simulink model "mixing_tank"  (R2019b)
settings: Solver=FixedStepDiscrete  StartTime=0.0  StopTime=30.0  FixedStep=1  RelTol=1e-3  EnableMultiTasking=on
undefined symbols (not defined in the file): sigbuilder_block
settings Model: EnablePacing=on  PacingRate=0.500000  Creator=faaizz  LastModifiedBy=faaizz
settings SolverCC: AutoInsertRateTranBlk=on
settings DataIOCC: LimitDataPoints=on
settings OptimizationCC: LifeSpan=inf
settings DebuggingCC: AllowSymbolicDim=off  SFUnexpectedBacktrackingDiag=warning  SFNoUnconditionalDefaultTransitionDiag=warning  SFExecutionAtInitializationDiag=none  ArithmeticOperatorsInVariantConditions=warning
settings SFSimCC: SimUseLocalCustomCode=off  CustomCodeUndefinedFunction=UseInterfaceOnly
settings RTWCC: RTWUseLocalCustomCode=off
settings CodeAppCC: StateflowObjectComments=on
settings GRTTargetCC: TargetLangStandard=C89/C90 (ANSI)  GeneratePreprocessorConditionals=Disable all
settings ConfigComp: CovMetricSettings=dw  CovHtmlReporting=on  CovSaveCumulativeToWorkspaceVar=on  CovSaveSingleToWorkspaceVar=on  CovShowResultsExplorer=off  CovExternalEMLEnable=off  CovSFcnEnable=off

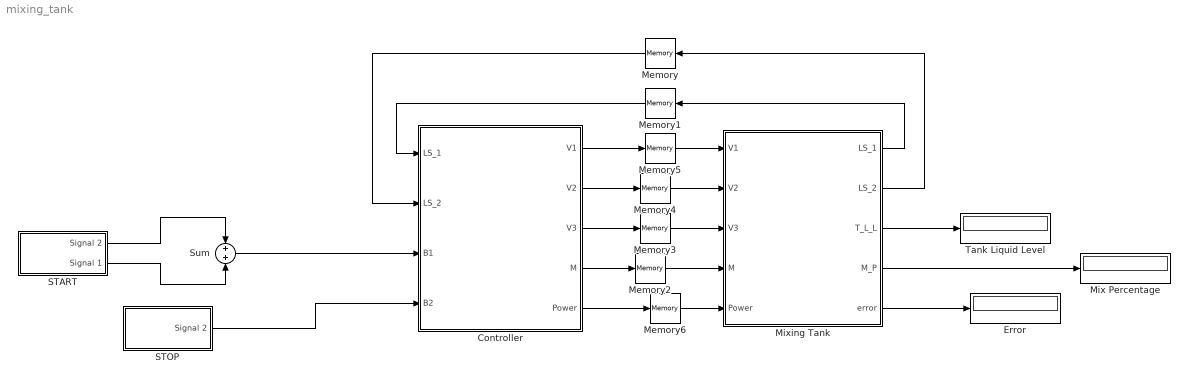
== system mixing_tank ==
  Controller : Stateflow chart  BlockKeywords=__PRM__SERIALIZED__DATA__:Stateflow Chart,Stateflow Diagram  TreatAsAtomicUnit=on
  Error : Display
  Memory{,1..6} (7 alike) : Memory
  Mix Percentage : Display
  Mixing Tank : Stateflow chart  TreatAsAtomicUnit=on
  START : Subsystem  Tag=STV Subsys  LoadFcn=sigbuilder_block('load');  StartFcn=sigbuilder_block('start');  StopFcn=sigbuilder_block('stop');  ClipboardFcn=sigbuilder_block('clipboard');  mask(Sigbuilder block){tuvar=[0:10]}
      mask help: Simulink:masks:SigbuilderBlock_MD
      mask init:
      | if ~strcmp(get_param(bdroot(gcbh),'SimulationStatus'),'stopped') tuvar = sigbuilder_block('maskInit'); end
      settings: CopyFcn=sigbuilder_block('copy');  DeleteFcn=sigbuilder_block('delete');  ModelCloseFcn=sigbuilder_block('modelClose');  PreSaveFcn=sigbuilder_block('preSave');  PauseFcn=sigbuilder_block('pause');  ContinueFcn=sigbuilder_block('continue');  NameChangeFcn=sigbuilder_block('namechange');  OpenFcn=sigbuilder_block('open',[278.25 69.75 628.5 342.75 ]);  CloseFcn=sigbuilder_block('close');
      mask Display: plot(0, 0, 100, 100,[2, 2, 32, 32, 2], [68, 8, 8, 68, 68],[32, 2], [38, 38], [32, 19, 2],[53, 60, 44], [32, 17, 17, 2],[16, 16, 31, 31]);txt = getActiveGroup(gcbh);text(2, 100, txt,'verticalAlignment', 'top');
  STOP : Subsystem  Tag=STV Subsys  LoadFcn=sigbuilder_block('load');  StartFcn=sigbuilder_block('start');  StopFcn=sigbuilder_block('stop');  ClipboardFcn=sigbuilder_block('clipboard');  mask(Sigbuilder block){tuvar=[0:10]}
      mask help: Simulink:masks:SigbuilderBlock_MD
      mask init:
      | if ~strcmp(get_param(bdroot(gcbh),'SimulationStatus'),'stopped') tuvar = sigbuilder_block('maskInit'); end
      settings: CopyFcn=sigbuilder_block('copy');  DeleteFcn=sigbuilder_block('delete');  ModelCloseFcn=sigbuilder_block('modelClose');  PreSaveFcn=sigbuilder_block('preSave');  PauseFcn=sigbuilder_block('pause');  ContinueFcn=sigbuilder_block('continue');  NameChangeFcn=sigbuilder_block('namechange');  OpenFcn=sigbuilder_block('open',[433.5 124.5 558 353.25 ]);  CloseFcn=sigbuilder_block('close');
      mask Display: plot(0, 0, 100, 100,[2, 2, 32, 32, 2], [68, 8, 8, 68, 68],[32, 2], [38, 38], [32, 19, 2],[53, 60, 44], [32, 17, 17, 2],[16, 16, 31, 31]);txt = getActiveGroup(gcbh);text(2, 100, txt,'verticalAlignment', 'top');
  Sum : Sum
  Tank Liquid Level : Display
  wires:
  Controller/5(Power) -> Memory6/1
  Controller/1(V1) -> Memory5/1
  Controller/2(V2) -> Memory4/1
  Controller/3(V3) -> Memory3/1
  Controller/4(M) -> Memory2/1
  Mixing Tank/1(LS_1) -> Memory1/1
  Mixing Tank/2(LS_2) -> Memory/1
  Mixing Tank/3(T_L_L) -> Tank Liquid Level/1
  Mixing Tank/4(M_P) -> Mix Percentage/1
  Mixing Tank/5(error) -> Error/1
  STOP/1(Signal 2) -> Controller/4(B2)
  Memory/1 -> Controller/2(LS_2)
  Memory1/1 -> Controller/1(LS_1)
  Memory5/1 -> Mixing Tank/1(V1)
  Memory4/1 -> Mixing Tank/2(V2)
  Memory3/1 -> Mixing Tank/3(V3)
  Memory2/1 -> Mixing Tank/4(M)
  Memory6/1 -> Mixing Tank/5(Power)
  Sum/1 -> Controller/3(B1)
  START/2(Signal 1) -> Sum/2
  START/1(Signal 2) -> Sum/1

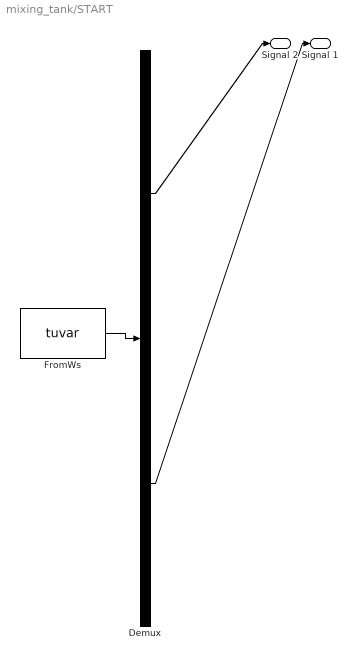
== system mixing_tank/START ==
  Demux : Demux  Tag=STV Demux  Outputs=2
  FromWs : FromWorkspace  Tag=STV FromWs  VariableName=tuvar  SampleTime=0
      SigBuilderData=|
      | common.afterFinalStr = 'Extrapolate'
      | common.sampleTime = 0
      | dataSet.timeRange = [0 20]
      | dataSet.name = 'Group 1'
      | sbobj.Groups.Name = 'Group 1'
      | sbobj.Groups.Signals(1).Name = 'Signal 2'
      | sbobj.Groups.Signals(1).XData = [0 1 1 2 2 20]
      | sbobj.Groups.Signals(1).YData = [0 0 1 1 0 0]
      | sbobj.Groups.Signals(2).Name = 'Signal 1'
      | sbobj.Groups.Signals(2).XData = [0 9 9 10 10 20]
      | sbobj.Groups.Signals(2).YData = [0 0 1 1 0 0]
      | sbobj.Groups.TimeRange = [0 20]
  Signal 2 : Outport  Tag=STV Outport
  Signal 1 : Outport  Tag=STV Outport  Port=2
  wires:
  FromWs/1 -> Demux/1
  Demux/1 -> Signal 2/1
  Demux/2 -> Signal 1/1

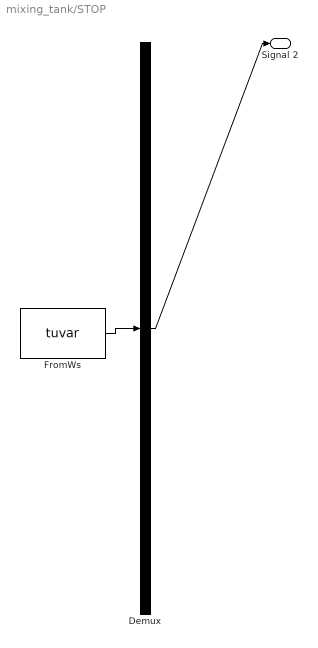
== system mixing_tank/STOP ==
  Demux : Demux  Tag=STV Demux  Outputs=1
  FromWs : FromWorkspace  Tag=STV FromWs  VariableName=tuvar  SampleTime=0
      SigBuilderData=|
      | common.afterFinalStr = 'Extrapolate'
      | common.sampleTime = 0
      | dataSet.timeRange = [0 10]
      | dataSet.name = 'Group 1'
      | sbobj.Groups.Name = 'Group 1'
      | sbobj.Groups.Signals.Name = 'Signal 2'
      | sbobj.Groups.Signals.XData = [0 6 6 8 8 10]
      | sbobj.Groups.Signals.YData = [0 0 1 1 0 0]
  Signal 2 : Outport  Tag=STV Outport
  wires:
  FromWs/1 -> Demux/1
  Demux/1 -> Signal 2/1

== stateflow chart mixing_tank/Controller ==
  state init
    % Entry
    entry:
    V1=0;
    V2=0;
    V3=0;
    M=0;
    Power=0;
    sus=0;
    % During
    during:
    V1=0;
    V2=0;
    V3=0;
    M=0;
    Power=0;
  state Stopped
    % Entry
    entry:
    V1=0;
    V2=0;
    V3=0;
    M=0;
    Power=1;
    % During
    V1=0;
    V2=0;
    V3=0;
    M=0;
    Power=1;
  state Filling
    % Entry
    entry:
    V1=1;
    V2=1;
    V3=0;
    M=0;
    Power=1;
    sus= 1;
    % During
    during:
    V1=1;
    V2=1;
    V3=0;
    M=0;
    Power=1;
  state Draining
    % Entry
    entry:
    V1=0;
    V2=0;
    V3=1;
    M=0;
    sus=3;
    Power=1;
    % During
    during:
    V1=0;
    V2=0;
    V3=1;
    M=0;
    Power=1;
  state Mixing
    % Entry
    entry:
    V1= 0;
    V2= 0;
    V3=0;
    M= 1;
    sus=2;
    T_10=0;
    Power=1;
    % During
    during:
    V1= 0;
    V2= 0;
    V3=0;
    M= 1;
    T_10= T_10+2;
    Power=1;
  (default) -> init
  init -> Mixing [order 2] : [B1== 1 & LS_2==1]
  init -> Filling [order 1] : [B1==1 & LS_2==0]
  Draining -> init [order 2] : [LS_1==0]
  Stopped -> Filling [order 1] : [B1== 1 & sus== 1]
  Draining -> Stopped [order 1] : [B2==1]
  Filling -> Stopped [order 1] : [B2==1]
  Stopped -> Draining [order 3] : [B1==1 & sus==3]
  Stopped -> Mixing [order 2] : [B1==1 & sus==1]
  Mixing -> Stopped [order 1] : [B2==1]
  Filling -> Mixing [order 2] : [LS_2 == 1]
  Mixing -> Draining [order 2] : [T_10>=10]
  data: LS_1 input; LS_2 input; B1 input; B2 input; V1 output; V2 output; V3 output; M output; sus local; Power output; T_10 local

== stateflow chart mixing_tank/Mixing Tank ==
  state eval_valves [function]
    (default) -> (junction 70) : % Valve 1
    (junction 70) -> (junction 71) [order 1] : [V1 == 1]
    (junction 70) -> (junction 72) [order 2]
    (junction 71) -> (junction 73) : {valve(1);}
    (junction 73) -> (junction 72)
    (junction 72) -> (junction 74)
    (junction 74) -> (junction 81) : % Valve 2
    (junction 81) -> (junction 82) [order 1] : [V2 == 1]
    (junction 81) -> (junction 83) [order 2]
    (junction 82) -> (junction 84) : {valve(1);}
    (junction 84) -> (junction 83)
    (junction 83) -> (junction 85)
    (junction 85) -> (junction 92) : % Valve 3
    (junction 92) -> (junction 93) [order 1] : [V3 == 1]
    (junction 92) -> (junction 94) [order 2]
    (junction 93) -> (junction 95) : {valve(-1);}
    (junction 95) -> (junction 94)
    (junction 94) -> (junction 96)
  state Off
  state valve(op) [function]
    (default) -> (junction 30) : % Perform valve operation
    (junction 30) -> (junction 31) [order 1] : [op < 0]
    (junction 30) -> (junction 32) [order 2] : {T_L_L= T_L_L+1;}
    (junction 31) -> (junction 33) : {T_L_L= T_L_L-1;}
    (junction 33) -> (junction 32)
    (junction 32) -> (junction 34)
    (junction 34) -> (junction 41)
    (junction 41) -> (junction 42) [order 1] : [T_L_L<0]
    (junction 41) -> (junction 43) [order 2]
    (junction 42) -> (junction 44) : {T_L_L= 0;}
    (junction 44) -> (junction 43)
    (junction 43) -> (junction 45)
    (junction 45) -> (junction 53)
    (junction 53) -> (junction 54) [order 1] : [T_L_L> 100]
    (junction 53) -> (junction 55) [order 2]
    (junction 54) -> (junction 56) : {T_L_L= 100;}
    (junction 56) -> (junction 55)
    (junction 55) -> (junction 57)
  state eval_mixer [function]
    (default) -> (junction 186) : % If there's no liquid to mix, raise an error
    (junction 186) -> (junction 190) [order 1] : [T_L_L >=  0]
    (junction 190) -> (junction 183) : % Mixer
    (junction 186) -> (junction 187) [order 2] : {error= 1;}
    (junction 183) -> (junction 180) [order 1] : [M == 1]
    (junction 183) -> (junction 184) [order 2]
    (junction 180) -> (junction 178) : {M_P= M_P+1.5;}
    (junction 178) -> (junction 184)
    (junction 184) -> (junction 119) : % Limit mixer percentage
    (junction 119) -> (junction 120) [order 1] : [M_P > 100]
    (junction 119) -> (junction 121) [order 2]
    (junction 120) -> (junction 122) : {M_P= 100;}
    (junction 122) -> (junction 121)
    (junction 121) -> (junction 123)
    (junction 187) -> (junction 123)
    (junction 123) -> (junction 195)
  state eval_output [function]
    (default) -> (junction 138) : % Empty Tank
    (junction 138) -> (junction 139) [order 1] : [T_L_L < 10]
    (junction 138) -> (junction 140) [order 2]
    (junction 139) -> (junction 141) : {LS_1= 0;}
    (junction 141) -> (junction 140)
    (junction 140) -> (junction 142)
    (junction 142) -> (junction 149) : % Full Tank
    (junction 149) -> (junction 150) [order 1] : [T_L_L > 95]
    (junction 149) -> (junction 151) [order 2]
    (junction 150) -> (junction 152) : {LS_2= 1;}
    (junction 152) -> (junction 151)
    (junction 151) -> (junction 153)
  state On
    % Entry
    entry:
    % Set all outputs defualts
    LS_1= 1;
    LS_2= 0;
    T_L_L= 0;
    M_P= 0;
    % During
    during:
    eval_valves
    eval_mixer
    eval_output
  (default) -> Off : {error=0}
  Off -> On : [Power == 1 & error==0]
  On -> Off : [Power==0 | error==1]
  data: op function_input; V1 input; V2 input; V3 input; M input; LS_1 output; LS_2 output; T_L_L output; M_P output; Power input; error output
